simulink model "IFFT_Ex2"  (R2023a)
settings: Solver=VariableStepAuto  StartTime=0.0  StopTime=2  RelTol=1e-3
undefined symbols (not defined in the file): None, S, vsva2197, xcvc1902
libraries: dspxfrm3 x2, aieDSP x1, aieUtilities x1, dspsrcs4 x1, vmcUtilities x1
settings Model: Creator=sdegala  LastModifiedBy=robg
settings ModelReferenceCC: EnableRefExpFcnMdlSchedulingChecks=on

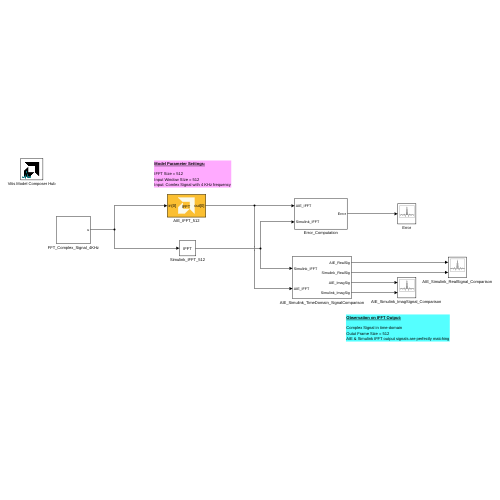
[thumbnail: Simulink's stored preview of the top-level diagram]
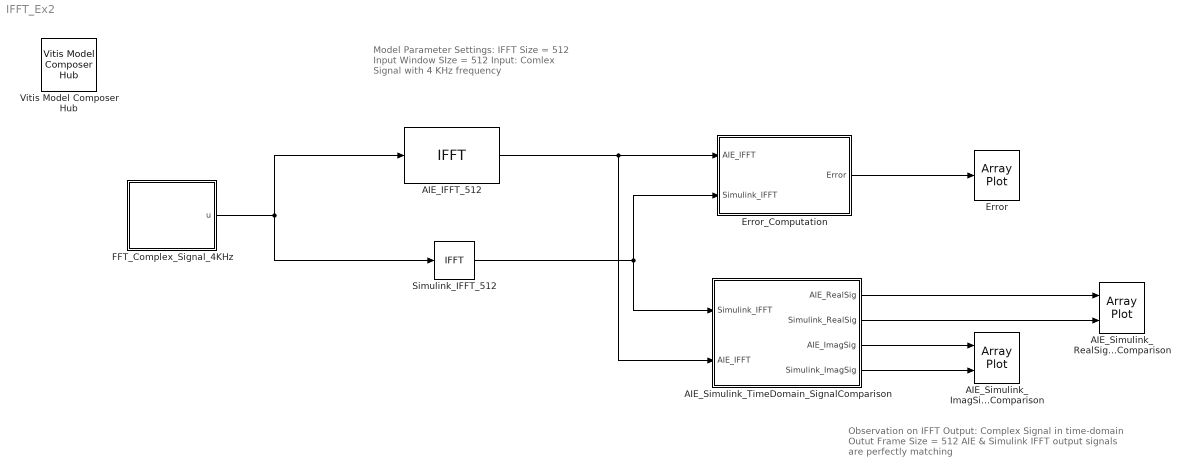
== system IFFT_Ex2 ==
  note: Model Parameter Settings:
      |
      | IFFT Size = 512
      | Input Window SIze = 512
      | Input: Comlex Signal with 4 KHz frequency
  note: Observation on IFFT Output:
      |
      | Complex Signal in time-domain
      | Outut Frame Size = 512
      | AIE & Simulink IFFT output signals are perfectly matching
  AIE_IFFT_512 : aieDSP/IFFT  data_type=cfloat  data_out_type=cfloat  twiddle_type=cfloat  point_size=512  input_window_size=512  shift_val=0  rnd_mode=Round symmetrical to infinity  sat_mode=0-None  ssr=1  twiddle_mode=0  use_ssr_widget_kernels=off  casc_length=1  AIE_VARIANT=1  blockJsonConstraints=[]  blockJsonConstraintsInternal=[]  spec=vmc_ifft.json  SerializedMaskParamNames=[]  SerializedMaskParamValues=[]  SerializedMaskParamVisibilities=[]  block_type=IFFT  SerializedMaskParamDataypes=typename|typename|typename|uint|uint|uint|uint|uint|uint|uint|bool|uint|uint  SerializedMaskParamEnumStrArr=0|0|0|0|0|0|Round to positive infinity,Round to negative infinity,Round symmetrical to infinity,Round symmetrical to zero,Round convergent to even,Round convergent to odd|0-None,1-Asymmetric,3-Symmetric|0|0|0|0|0  SerializedMaskParamEnumValArr=0|0|0|0|0|0|2,3,4,5,6,7|0,1,3|0|0|0|0|0  SerializedMaskParamVectorArr=0|0|0|0|0|0|0|0|0|0|0|0|0
  "AIE_Simulink_ImagSignal_Comparison " : ArrayPlot  NumInputPorts=2  WindowPosition=[5.000000,269.000000,845.000000,423.000000,]  PlotType=Line  YLimits=[-0.0001,0]  ShowLegend=on
  AIE_Simulink_RealSignal_Comparison : ArrayPlot  NumInputPorts=2  WindowPosition=[2.000000,37.000000,1280.000000,655.000000,]  PlotType=Line  YLimits=[-1280,1280]  ShowLegend=on
  AIE_Simulink_TimeDomain_SignalComparison : Subsystem
  Error : ArrayPlot  WindowPosition=[338.000000,41.000000,800.000000,500.000000,]  XDataMode=Custom  PlotType=Line  ShowLegend=on
  Error_Computation : Subsystem
  FFT_Complex_Signal_4KHz : Subsystem
  Simulink_IFFT_512 : dspxfrm3/IFFT  FFTImplementation=Auto  CompMethod=Table lookup  TableOpt=NEW  TableOptActive=Speed  BitRevOrder=off  cs_in=off  Normalize=off  InheritFFTLength=off  FFTLength=512  WrapInput=on  mode=Complex  outSamplingMode=Sample based  roundingMode=Floor  overflowMode=off  firstCoeffDataTypeStr=Inherit: Same word length as input  firstCoeffLastDataTypeStr=Inherit: Same word length as input  outputMin=[]  outputMax=[]
  Vitis Model Composer Hub : vmcUtilities/Vitis Model Composer Hub  Tag=genX  CodeGeneration=off  StartColumn=1  NumberOfColumns=1  TargetDirectory=./code  exportDesign=off  analyzeDesign=off  validateDesignOnHw=off  ExportType=AI Engines  IpVendor=xilinx.com  IpLibrary=hls  IpVersion=1.0  IpHWLanguage=Verilog  AieCompilerOptions={}  AieSimulatorOptions={}  CreateTestbench=off  TestbenchStackSize=10  RunRtlSim=off  RunCSim=off  RunAieSim=off  AieSimTimeout=50000  RunAieSimProfiling=off  LaunchVitisAnalyzer=off  PlotOutput=off  RunX86Sim=off  X86SimTimeout=10  GenHwImage=off  GenLibadfXo=off  GenHwValidationCode=off  PlatformType=Not Specified  HwSystemType=Baremetal  HwValidationTarget=hw  ProjDevice=xcvc1902-vsva2197-1LP-e-S  ProjDevicePart=xcvc1902-vsva2197-1LP-e-S  AIEType=AIE  SamplePeriod=-1  ClockFrequency=200  DataPathParallelism=1  xilinxfamily=versalaicore  part=xcvc1902  speed=-1LP-e-S  package=vsva2197  directory=./netlist  testbench=off  incr_netlist=off  synthesis_tool=Vivado  clock_wrapper=Clock Enables  dbl_ovrd=According to Block Masks  dcm_input_clock_period=10  sysclk_period=10  simulink_period=1  eval_field=0  LogFileName=''  NThreads=4
  wires:
  AIE_Simulink_TimeDomain_SignalComparison/1(AIE_RealSig) -> AIE_Simulink_RealSignal_Comparison/1
  Simulink_IFFT_512/1 -> Error_Computation/2(Simulink_IFFT), AIE_Simulink_TimeDomain_SignalComparison/1(Simulink_IFFT)
  Error_Computation/1(Error) -> Error/1
  AIE_IFFT_512/1 -> AIE_Simulink_TimeDomain_SignalComparison/2(AIE_IFFT), Error_Computation/1(AIE_IFFT)
  AIE_Simulink_TimeDomain_SignalComparison/2(Simulink_RealSig) -> AIE_Simulink_RealSignal_Comparison/2
  FFT_Complex_Signal_4KHz/1(u) -> AIE_IFFT_512/1, Simulink_IFFT_512/1
  AIE_Simulink_TimeDomain_SignalComparison/4(Simulink_ImagSig) -> "AIE_Simulink_ImagSignal_Comparison "/2
  AIE_Simulink_TimeDomain_SignalComparison/3(AIE_ImagSig) -> "AIE_Simulink_ImagSignal_Comparison "/1

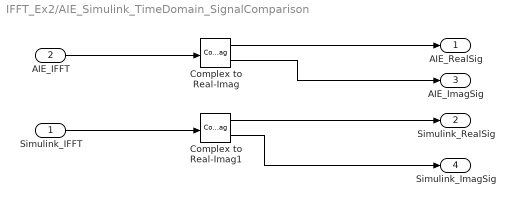
== system IFFT_Ex2/AIE_Simulink_TimeDomain_SignalComparison ==
  Simulink_IFFT : Inport
  AIE_IFFT : Inport  Port=2
  Complex to Real-Imag : ComplexToRealImag
  Complex to Real-Imag1 : ComplexToRealImag
  AIE_RealSig : Outport
  Simulink_RealSig : Outport  Port=2
  AIE_ImagSig : Outport  Port=3
  Simulink_ImagSig : Outport  Port=4
  wires:
  AIE_IFFT/1 -> Complex to Real-Imag/1
  Complex to Real-Imag/1 -> AIE_RealSig/1
  Complex to Real-Imag1/1 -> Simulink_RealSig/1
  Complex to Real-Imag1/2 -> Simulink_ImagSig/1
  Complex to Real-Imag/2 -> AIE_ImagSig/1
  Simulink_IFFT/1 -> Complex to Real-Imag1/1

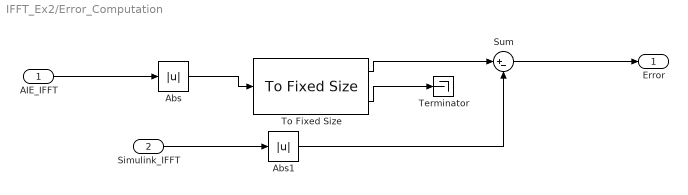
== system IFFT_Ex2/Error_Computation ==
  AIE_IFFT : Inport
  Simulink_IFFT : Inport  Port=2
  Abs : Abs  SaturateOnIntegerOverflow=off
  Abs1 : Abs  SaturateOnIntegerOverflow=off
  Sum : Sum  Inputs=|+-
  Terminator : Terminator
  To Fixed Size : aieUtilities/To Fixed Size  Mode=Produce a valid output signal  OutputSize=512*1  CopyMethod=Buffer samples to form output  HasStatusOutput=on
  Error : Outport
  wires:
  Abs1/1 -> Sum/2
  Simulink_IFFT/1 -> Abs1/1
  AIE_IFFT/1 -> Abs/1
  Sum/1 -> Error/1
  To Fixed Size/2 -> Terminator/1
  Abs/1 -> To Fixed Size/1
  To Fixed Size/1 -> Sum/1

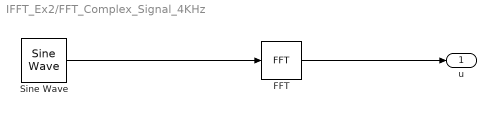
== system IFFT_Ex2/FFT_Complex_Signal_4KHz ==
  FFT : dspxfrm3/FFT  FFTImplementation=Auto  CompMethod=Table lookup  TableOpt=NEW  TableOptActive=Speed  BitRevOrder=off  Normalize=off  InheritFFTLength=off  FFTLength=512  WrapInput=on  roundingMode=Floor  overflowMode=off  firstCoeffDataTypeStr=Inherit: Same word length as input  firstCoeffLastDataTypeStr=Inherit: Same word length as input  outputMin=[]  outputMax=[]
  Sine Wave : dspsrcs4/Sine Wave  Amplitude=2  Frequency=4e3  Phase=0  SampleMode=Discrete  OutComplex=Complex  CompMethod=Trigonometric fcn  TableSize=Speed  SampleTime=1/8e3  SamplesPerFrame=512  ResetState=Restart at time zero  OutputFrames=off  dataType=single  wordLen=16  udDataType=sfix(16)  fracBitsMode=Best precision  numFracBits=15  OutDataTypeStr=single  LastOutDataTypeStr=single
  u : Outport
  wires:
  Sine Wave/1 -> FFT/1
  FFT/1 -> u/1
